simulink model "problem3"  (R2020b)
settings: Solver=VariableStepAuto  StartTime=0.0  StopTime=1  MaxStep=0.01  RelTol=1e-3
settings Model: Creator=k.Raviteja  LastModifiedBy=k.Raviteja

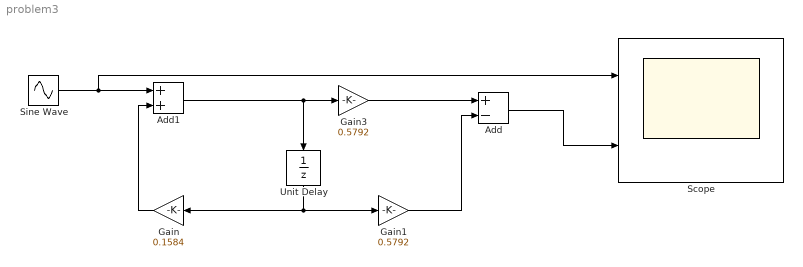
== system problem3 ==
  Add : Sum  Inputs=+-
  Add1 : Sum
  Gain : Gain  Gain=0.1584
  Gain1 : Gain  Gain=0.5792
  Gain3 : Gain  Gain=0.5792
  Scope : Scope  NumInputPorts=2
  Sine Wave : Sin  Frequency=1000  SampleTime=0
  Unit Delay : UnitDelay  SampleTime=-1  HasFrameUpgradeWarning=on
  wires:
  Unit Delay/1 -> Gain1/1, Gain/1
  Gain1/1 -> Add/2
  Gain/1 -> Add1/2
  Sine Wave/1 -> Scope/1, Add1/1
  Add1/1 -> Gain3/1, Unit Delay/1
  Gain3/1 -> Add/1
  Add/1 -> Scope/2
